simulink model "PneumaticsSystem"  (R2019b)
settings: configuration reference "ConfigSet_PneumaticsSystem_Reference" (kept outside this file)
PostLoadFcn:
  | set_up_test_model()
model workspace (MAT data in the model file):
  PAtm = 101300
  Prm_PneumaticsSystem = Simulink.Parameter
  Prm_PneumaticsSystem.Value.BrakeControl.LoadCompensationGains = [0.66 1]
  Prm_PneumaticsSystem.Value.BrakeControl.MaxPressure = 443000
  Prm_PneumaticsSystem.Value.MainReservoir.ResetPressure = 1000000
  Prm_PneumaticsSystem.Value.MainReservoir.MaxPressure = 1200000
  Prm_PneumaticsSystem.Value.MainReservoir.Volume = 0.2
  Prm_PneumaticsSystem.Value.MainReservoir.SwitchONPressure = 1000000
  Prm_PneumaticsSystem.Value.MainReservoir.SwitchOFFPressure = 750000
  Prm_PneumaticsSystem.Value.MainReservoir.CompressorMassFlowRate = 0.022
  Prm_PneumaticsSystem.Value.MainReservoir.BlowOffONPressure = 1050000
  Prm_PneumaticsSystem.Value.MainReservoir.BlowOffOFFPressure = 1000000
  Prm_PneumaticsSystem.Value.MainReservoirPipe.ResetPressure = 1000000
  Prm_PneumaticsSystem.Value.MainReservoirPipe.SwitchONPressure = 1000000
  Prm_PneumaticsSystem.Value.MainReservoirPipe.SwitchOFFPressure = 750000
  Prm_PneumaticsSystem.Value.Sanding.SwitchONPressure = 380000
  Prm_PneumaticsSystem.Value.Sanding.SwitchOFFPressure = 360000
  Prm_PneumaticsSystem.Value.AirSuspension.LoadCompensationMasses = [21000 33350]
  Prm_PneumaticsSystem.Value.AirSuspension.LoadCompensationPressures = [165000 440000]
  Prm_PneumaticsSystem.Value.AirSuspension.MaxPressure = 510000
  Prm_PneumaticsSystem.Value.AirSuspension.Volume = 0.07
  Prm_PneumaticsSystem.Value.AirSuspension.SwitchONPressure = 220000
  Prm_PneumaticsSystem.Value.AirSuspension.SwitchOFFPressure = 180000
  Prm_PneumaticsSystem.Value.Horn.SwitchONPressure = 140000
  Prm_PneumaticsSystem.Value.AuxiliaryReservoir.ResetPressure = 1000000
  Prm_PneumaticsSystem.Value.AuxiliaryReservoir.MaxPressure = 1000000
  Prm_PneumaticsSystem.Value.AuxiliaryReservoir.Volume = 0.025
  Prm_PneumaticsSystem.Value.AuxiliaryReservoir.SwitchONPressure = 700000
  Prm_PneumaticsSystem.Value.AuxiliaryReservoir.SwitchOFFPressure = 600000
  Prm_PneumaticsSystem.Value.AuxiliaryReservoir.CompressorMassFlowRate = 0.0014
  Prm_PneumaticsSystem.Value.AuxiliaryReservoir.BlowOffONPressure = 1020000
  Prm_PneumaticsSystem.Value.AuxiliaryReservoir.BlowOffOFFPressure = 1000000
  Prm_PneumaticsSystem.Value.Pantograph.ResetPressure = 0
  Prm_PneumaticsSystem.Value.Pantograph.MaxPressure = 1000000
  Prm_PneumaticsSystem.Value.Pantograph.Volume = 0.003
  Prm_PneumaticsSystem.Value.Pantograph.SwitchONPressure = 380000
  Prm_PneumaticsSystem.Value.Pantograph.SwitchOFFPressure = 280000
  Prm_PneumaticsSystem.Value.Pantograph.ORDSwitchONPressure = 300000
  Prm_PneumaticsSystem.Value.Pantograph.ORDSwitchOFFPressure = 240000
  Prm_PneumaticsSystem.Value.BrakeReservoir.ResetPressure = 1000000
  Prm_PneumaticsSystem.Value.BrakeReservoir.MaxPressure = 1200000
  Prm_PneumaticsSystem.Value.BrakeReservoir.Volume = 0.1
  Prm_PneumaticsSystem.Value.BrakeReservoir.SwitchONPressure = 650000
  Prm_PneumaticsSystem.Value.BrakeReservoir.SwitchOFFPressure = 550000
  Prm_PneumaticsSystem.Value.BrakeCylinder.BrakeCylindersPerBogieAxle = [2 2]
  Prm_PneumaticsSystem.Value.BrakeCylinder.ResetPressure = 0
  Prm_PneumaticsSystem.Value.BrakeCylinder.MaxPressure = 600000
  Prm_PneumaticsSystem.Value.BrakeCylinder.Volume = 0.0125
  Prm_PneumaticsSystem.Value.BrakeCylinder.SwitchONPressure = 60000
  Prm_PneumaticsSystem.Value.BrakeCylinder.SwitchOFFPressure = 30000
  Prm_PneumaticsSystem.Value.ParkBrakes.ParkBrakesPerBogieAxle = [1 1]
  Prm_PneumaticsSystem.Value.ParkBrakes.ParkBrakePressures = [300000 480000]
  Prm_PneumaticsSystem.Value.ParkBrakes.ParkBrakeForces = [31500 0]
  Prm_PneumaticsSystem.Value.ParkBrakes.SwitchONPressure = 480000
  Prm_PneumaticsSystem.Value.ParkBrakes.SwitchOFFPressure = 380000
  Prm_PneumaticsSystem.Value.VCB.ResetPressure = 0
  Prm_PneumaticsSystem.Value.VCB.MaxPressure = 1000000
  Prm_PneumaticsSystem.Value.VCB.Volume = 0.0005
  Prm_PneumaticsSystem.Value.VCB.SwitchONPressure = 435000
  Prm_PneumaticsSystem.Value.VCB.SwitchOFFPressure = 385000
  Prm_PneumaticsSystem.DataType = 'Bus: BD_PneumaticsSystem_Prm'
  Prm_PneumaticsSystem.Dimensions = [1 1]
  SampleTime = 0.01
undefined symbols (not defined in the file): AirSuspensionBogie1Deflated, AirSuspensionPressure, AirSuspensionPressureSwitch, AirSuspPressureDiff, AuxiliaryReservoirPressure, AuxiliaryReservoirPressureSwitch, BECU1BrakeNotApplied, BECU1BrakeNotReleased, BECU1CarLoadPressureLow, BECU1EmergencyBrakeFailure, BECU1LoadPressureLow, BECU1ServiceBrakeFailure, BECU2CarLoadPressureLow, BECU2EmergencyBrakeFailure, BECULowRPressure, Bogie, BrakeCylinderControlPressure, BrakeCylinderPressure, BrakeCylinderPressureGauge, BrakeCylinderPressureSwitch, BrakeReservoirPressure, BrakeReservoirPressureSwitch, HornHighPressureSwitch, HornLowPressureSwitch, MainReservoirPipePressure, MainReservoirPipePressureSwitch, MainReservoirPressure, MainReservoirPressureGauge, MainReservoirPressureSwitch, MaxAxles, MRPS_TractionCutout, ORDPressureSwitch, PantographCylinderPressure, ParkBrakePressure, ParkBrakePressureGauge, ParkBrakePressureSwitch, PS2, PS3, SandingSystemPressure, SandingSystemPressureSwitch, SRPressureGauge, VCBCylinderPressure, VCBPressureSwitch
libraries: PneumaticLib x56, simulink x50, LatchesLib x7, FiltersLib x4, TimersLib x3, MathOperationsLib x3, VectorOperationsLib x1, simulink_extras x1
(part 1 of 3)
settings Model: PauseTimes=3  ParameterArgumentNames=Prm_PneumaticsSystem  Creator=cdyer  LastModifiedBy=hinganes
settings ConfigSetRef: SourceName=ConfigSet_PneumaticsSystem_Reference  SourceLocation=Base Workspace

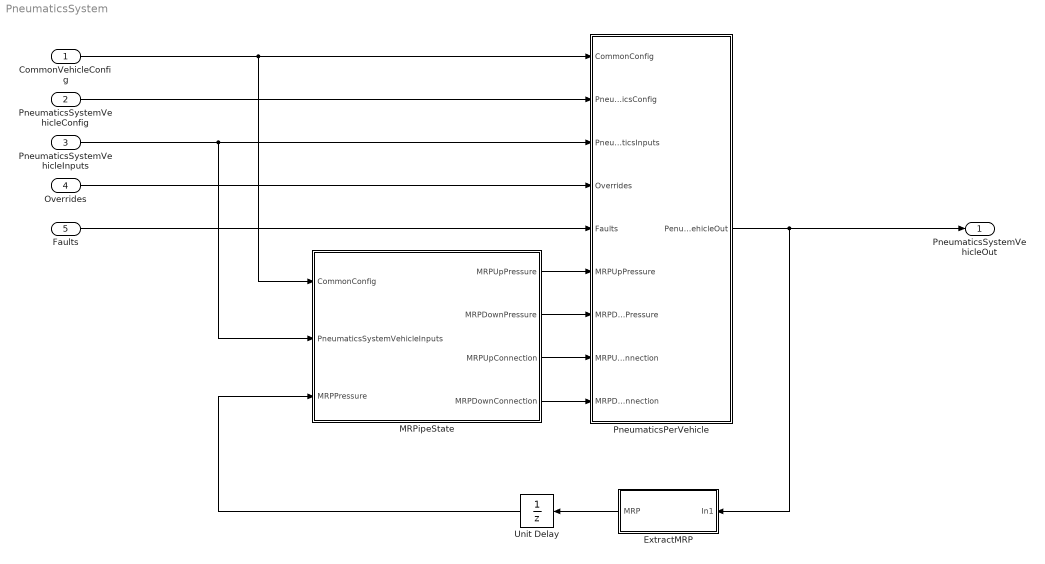
== system PneumaticsSystem ==
  CommonVehicleConfig : Inport  OutDataTypeStr=Bus: BD_CommonTrain_Cfg_Vehicle  PortDimensions=MaxVehicles  BusOutputAsStruct=on
  PneumaticsSystemVehicleConfig : Inport  Port=2  OutDataTypeStr=Bus: BD_PneumaticsSystem_Cfg_Vehicle  PortDimensions=MaxVehicles  BusOutputAsStruct=on
  PneumaticsSystemVehicleInputs : Inport  Port=3  OutDataTypeStr=Bus: BD_PneumaticsSystem_In_Vehicle  PortDimensions=MaxVehicles  BusOutputAsStruct=on
  Overrides : Inport  Port=4  OutDataTypeStr=Bus: BD_PneumaticsSystem_In_Overrides  BusOutputAsStruct=on
  Faults : Inport  Port=5  OutDataTypeStr=Bus: BD_PneumaticsSystem_In_Vehicle_Faults  BusOutputAsStruct=on
  ExtractMRP : Subsystem  TreatAsAtomicUnit=on
  MRPipeState : Subsystem
  PneumaticsPerVehicle : Subsystem
  Unit Delay : UnitDelay  SampleTime=-1  HasFrameUpgradeWarning=on
  PneumaticsSystemVehicleOut : Outport  OutDataTypeStr=Bus: BD_PneumaticsSystem_Out_Vehicle  BusOutputAsStruct=on
  wires:
  Faults/1 -> PneumaticsPerVehicle/5(Faults)
  PneumaticsSystemVehicleInputs/1 -> PneumaticsPerVehicle/3(PneumaticsInputs), MRPipeState/2(PneumaticsSystemVehicleInputs)
  Overrides/1 -> PneumaticsPerVehicle/4(Overrides)
  PneumaticsPerVehicle/1(PenumaticsVehicleOut) -> PneumaticsSystemVehicleOut/1, ExtractMRP/1(In1)
  ExtractMRP/1(MRP) -> Unit Delay/1
  Unit Delay/1 -> MRPipeState/3(MRPPressure)
  MRPipeState/1(MRPUpPressure) -> PneumaticsPerVehicle/6(MRPUpPressure)
  MRPipeState/2(MRPDownPressure) -> PneumaticsPerVehicle/7(MRPDownPressure)
  MRPipeState/3(MRPUpConnection) -> PneumaticsPerVehicle/8(MRPUpConnection)
  CommonVehicleConfig/1 -> MRPipeState/1(CommonConfig), PneumaticsPerVehicle/1(CommonConfig)
  PneumaticsSystemVehicleConfig/1 -> PneumaticsPerVehicle/2(PneumaticsConfig)
  MRPipeState/4(MRPDownConnection) -> PneumaticsPerVehicle/9(MRPDownConnection)

== system PneumaticsSystem/ExtractMRP ==
  In1 : Inport  Partition=on  PartitionDimension=1  PartitionWidth=1  PartitionOffset=0
  Bus Selector1 : BusSelector  OutputSignals=Debug.MainReservoirPipePressure
  For Each : ForEach  DisableCoverage=on
  MRP : Outport  ConcatenationDimension=1
  wires:
  In1/1 -> Bus Selector1/1
  Bus Selector1/1 -> MRP/1  "<MainReservoirPipePressure>"

== system PneumaticsSystem/MRPipeState ==
  CommonConfig : Inport
  PneumaticsSystemVehicleInputs : Inport  Port=2
  MRPPressure : Inport  Port=3
  Extract : Subsystem  TreatAsAtomicUnit=on
  Head : Selector  NumberOfDimensions=2  InputPortWidth=3  IndexOptions=Select all,Index vector (dialog)  Indices=[1],[1]  OutputSizes=1,1
  Orientation Swap : VectorOperationsLib/Orientation Swap
      settings: SourceProductName=Sydac Utilities
  PipeConnections : MATLAB Function  TreatAsAtomicUnit=on
  Product : Product
  Product1 : Product
  Tail : Selector  NumberOfDimensions=2  InputPortWidth=3  IndexOptions=Select all,Index vector (dialog)  Indices=[1],[2]  OutputSizes=1,1
  UpDnSel : MATLAB Function  TreatAsAtomicUnit=on
  MRPUpPressure : Outport
  MRPDownPressure : Outport  Port=2
  MRPUpConnection : Outport  Port=3
  MRPDownConnection : Outport  Port=4
  wires:
  UpDnSel/2(yDn) -> MRPDownPressure/1
  MRPPressure/1 -> UpDnSel/1(u)
  UpDnSel/1(yUp) -> MRPUpPressure/1
  PipeConnections/2(rearState) -> MRPDownConnection/1
  PipeConnections/1(frontState) -> MRPUpConnection/1
  PneumaticsSystemVehicleInputs/1 -> Extract/2(PneumaticsSystemVehicleInputs)
  CommonConfig/1 -> Extract/1(CommonConfig)
  Extract/4(Orientation) -> Orientation Swap/3
  Orientation Swap/1 -> PipeConnections/1(frontCock)  "Front"
  Orientation Swap/2 -> PipeConnections/2(rearCock)  "Rear"
  Product/1 -> Orientation Swap/1
  Product1/1 -> Orientation Swap/2
  Extract/1(Enabled) -> Product1/1, Product/1
  Extract/2(End1Cock) -> Product/2
  Extract/3(End2Cock) -> Product1/2
  Head/1 -> PipeConnections/3(frontCoupled)  "Front"
  Tail/1 -> PipeConnections/4(rearCoupled)  "Rear"
  Extract/5(PneumaticCouplingState) -> Tail/1, Head/1

== system PneumaticsSystem/PneumaticsPerVehicle ==
  CommonConfig : Inport  Partition=on  PartitionDimension=1  PartitionWidth=1  PartitionOffset=0
  PneumaticsConfig : Inport  Port=2  Partition=on  PartitionDimension=1  PartitionWidth=1  PartitionOffset=0
  PneumaticsInputs : Inport  Port=3  Partition=on  PartitionDimension=1  PartitionWidth=1  PartitionOffset=0
  Overrides : Inport  Port=4  Partition=on  PartitionDimension=1  PartitionWidth=1  PartitionOffset=0
  Faults : Inport  Port=5  Partition=on  PartitionDimension=1  PartitionWidth=1  PartitionOffset=0
  MRPUpPressure : Inport  Port=6  Partition=on  PartitionDimension=1  PartitionWidth=1  PartitionOffset=0
  MRPDownPressure : Inport  Port=7  Partition=on  PartitionDimension=1  PartitionWidth=1  PartitionOffset=0
  MRPUpConnection : Inport  Port=8  Partition=on  PartitionDimension=1  PartitionWidth=1  PartitionOffset=0
  MRPDownConnection : Inport  Port=9  Partition=on  PartitionDimension=1  PartitionWidth=1  PartitionOffset=0
  Bus Selector : BusSelector  OutputSignals=Enabled
  For Each : ForEach  DisableCoverage=on
  PneumaticsSystem : Subsystem
  PenumaticsVehicleOut : Outport  ConcatenationDimension=1
  wires:
  CommonConfig/1 -> PneumaticsSystem/1(CommonConfig), Bus Selector/1
  PneumaticsInputs/1 -> PneumaticsSystem/3(PneumaticsInputs)
  Overrides/1 -> PneumaticsSystem/4(Overrides)
  Faults/1 -> PneumaticsSystem/5(Faults)
  MRPUpPressure/1 -> PneumaticsSystem/6(MRPUpPressure)
  MRPDownPressure/1 -> PneumaticsSystem/7(MRPDownPressure)
  MRPUpConnection/1 -> PneumaticsSystem/8(MRPUpConnection)
  MRPDownConnection/1 -> PneumaticsSystem/9(MRPDownConnection)
  PneumaticsSystem/1(PenumaticsVehicleOut) -> PenumaticsVehicleOut/1
  PneumaticsConfig/1 -> PneumaticsSystem/2(PneumaticsConfig)  "Pneumatics"
  Bus Selector/1 -> PneumaticsSystem/Enable  "<Enabled>"

== system PneumaticsSystem/MRPipeState/Extract ==
  CommonConfig : Inport  Partition=on  PartitionDimension=1  PartitionWidth=1  PartitionOffset=0
  PneumaticsSystemVehicleInputs : Inport  Port=2  Partition=on  PartitionDimension=1  PartitionWidth=1  PartitionOffset=0
  Bus Selector : BusSelector  OutputSignals=InputControlStates.InterCarIsolationCockEnd1,InputControlStates.InterCarIsolationCockEnd2,PhysicalSignals.PneumaticallyCoupled,InputControlStates.UncouplingIsolationCock
  Bus Selector2 : BusSelector  OutputSignals=Orientation,Enabled
  For Each : ForEach  DisableCoverage=on
  Logical Operator : Logic  AllPortsSameDT=off  OutDataTypeStr=boolean
  Reshape : Reshape  OutputDimensionality=Row vector (2-D)
  Enabled : Outport  ConcatenationDimension=1
  End1Cock : Outport  Port=2  ConcatenationDimension=1
  End2Cock : Outport  Port=3  ConcatenationDimension=1
  Orientation : Outport  Port=4  ConcatenationDimension=1
  PneumaticCouplingState : Outport  Port=5  ConcatenationDimension=1
  wires:
  CommonConfig/1 -> Bus Selector2/1
  Bus Selector2/1 -> Orientation/1  "<Orientation>"
  Bus Selector2/2 -> Enabled/1  "<Enabled>"
  PneumaticsSystemVehicleInputs/1 -> Bus Selector/1
  Bus Selector/1 -> End1Cock/1  "<InterCarIsolationCockEnd1>"
  Bus Selector/2 -> End2Cock/1  "<InterCarIsolationCockEnd2>"
  Bus Selector/3 -> Logical Operator/1  "<PneumaticallyCoupled>"
  Reshape/1 -> PneumaticCouplingState/1
  Bus Selector/4 -> Logical Operator/2  "<UncouplingIsolationCock>"
  Logical Operator/1 -> Reshape/1

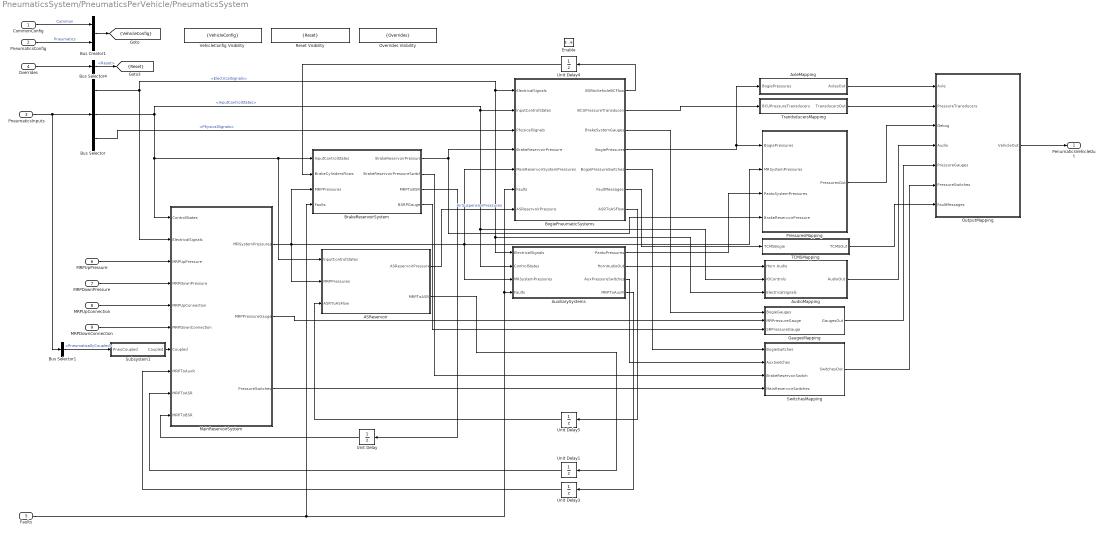
== system PneumaticsSystem/PneumaticsPerVehicle/PneumaticsSystem ==
  CommonConfig : Inport
  PneumaticsConfig : Inport  Port=2
  PneumaticsInputs : Inport  Port=3
  Overrides : Inport  Port=4
  Faults : Inport  Port=5
  MRPUpPressure : Inport  Port=6
  MRPDownPressure : Inport  Port=7
  MRPUpConnection : Inport  Port=8
  MRPDownConnection : Inport  Port=9
  Enable : EnablePort
  ASReservoir : Subsystem
  AudioMapping : Subsystem
  AuxiliarySystems : Subsystem
  AxleMapping : Subsystem
  BogiePneumaticSystems : Subsystem
  BrakeReservoirSystem : Subsystem
  Bus Creator1 : BusCreator  Inputs=2
  Bus Selector : BusSelector  OutputSignals=ElectricalSignals,InputControlStates,PhysicalSignals
  Bus Selector1 : BusSelector  OutputSignals=PhysicalSignals.PneumaticallyCoupled
  Bus Selector4 : BusSelector  OutputSignals=Reset
  GaugesMapping : Subsystem
  MainReservoirSystem : Subsystem
  OutputMapping : Subsystem
  Overrides Visibility : GotoTagVisibility  GotoTag=Overrides
  PressuresMapping : Subsystem
  Reset Visibility : GotoTagVisibility  GotoTag=Reset
  Subsystem1 : Subsystem
  SwitchesMapping : Subsystem
  TCMSMapping : Subsystem
  TrandsducersMapping : Subsystem
  Unit Delay{,1,3..5} (5 alike) : UnitDelay  SampleTime=-1  HasFrameUpgradeWarning=on
  VehicleConfig Visibility : GotoTagVisibility  GotoTag=VehicleConfig
  PenumaticsVehicleOut : Outport
  tag scope: Reset=scoped, VehicleConfig=scoped
  wires:
  Overrides/1 -> Bus Selector4/1
  OutputMapping/1(VehicleOut) -> PenumaticsVehicleOut/1
  AuxiliarySystems/1(PantoPressures) -> PressuresMapping/3(PantoSystemPressures)
  PneumaticsInputs/1 -> Bus Selector1/1, Bus Selector/1
  Bus Selector/1 -> AudioMapping/3(ElectricalSignals), AuxiliarySystems/1(ElectricalSignals), BogiePneumaticSystems/1(ElectricalSignals), MainReservoirSystem/2(ElectricalSignals)  "<ElectricalSignals>"
  Bus Selector/2 -> AudioMapping/2(IOControls), AuxiliarySystems/2(ControlStates), BogiePneumaticSystems/2(InputControlStates), MainReservoirSystem/1(ControlStates), ASReservoir/1(InputControlStates), BrakeReservoirSystem/1(InputControlStates)  "<InputControlStates>"
  Unit Delay/1 -> MainReservoirSystem/10(MRPToBSR)
  MRPUpPressure/1 -> MainReservoirSystem/3(MRPUpPressure)
  MRPDownPressure/1 -> MainReservoirSystem/4(MRPDownPressure)
  MRPUpConnection/1 -> MainReservoirSystem/5(MRPUpConnection)
  MRPDownConnection/1 -> MainReservoirSystem/6(MRPDownConnection)
  MainReservoirSystem/2(MRPPressureGauge) -> GaugesMapping/2(MRPressureGauge)
  PressuresMapping/1(PressuresOut) -> OutputMapping/3(Debug)
  GaugesMapping/1(GaugesOut) -> OutputMapping/5(PressureGauges)
  SwitchesMapping/1(SwitchesOut) -> OutputMapping/6(PressureSwitches)
  AudioMapping/1(AudioOut) -> OutputMapping/4(Audio)
  TrandsducersMapping/1(TransducersOut) -> OutputMapping/2(PressureTransducers)
  BrakeReservoirSystem/1(BrakeReservoirPressure) -> BogiePneumaticSystems/4(BrakeReservoirPressure), PressuresMapping/4(BrakeReservoirPressure)
  MainReservoirSystem/3(PressureSwitches) -> SwitchesMapping/4(MainReservoirSwitches)
  PneumaticsConfig/1 -> Bus Creator1/2  "Pneumatics"
  Bus Creator1/1 -> [VehicleConfig]
  Bus Selector4/1 -> [Reset]  "<Reset>"
  Bus Selector/3 -> BogiePneumaticSystems/3(PhysicalSignals)  "<PhysicalSignals>"
  AuxiliarySystems/2(HornAudioOut) -> AudioMapping/1(Horn Audio)
  AuxiliarySystems/3(AuxPressureSwitches) -> SwitchesMapping/2(AuxSwitches)
  Unit Delay3/1 -> MainReservoirSystem/8(MRPToAuxR)
  BogiePneumaticSystems/2(BCUPressureTransducers) -> TrandsducersMapping/1(BCUPressureTransducers)
  BogiePneumaticSystems/3(BrakeSystemGauges) -> GaugesMapping/1(BogieGauges)
  BogiePneumaticSystems/4(BogiePressures) -> AxleMapping/1(BogiePressures), PressuresMapping/1(BogiePressures)
  BogiePneumaticSystems/5(BogiePressureSwitches) -> SwitchesMapping/1(BogieSwitches)
  MainReservoirSystem/1(MRSystemPressures) -> BrakeReservoirSystem/3(MRPPressures), ASReservoir/2(MRPPressures), BogiePneumaticSystems/5(MainReservoirSystemPressures), PressuresMapping/2(MRSystemPressures), AuxiliarySystems/3(MRSystemPressures)
  BogiePneumaticSystems/1(BSRtoVehicleBCFlow) -> Unit Delay4/1
  Unit Delay4/1 -> BrakeReservoirSystem/2(BrakeCylindersFlows)
  ASReservoir/1(ASReservoirPressure) -> BogiePneumaticSystems/7(ASReservoirPressure)  "AirSuspensionPressures"
  BrakeReservoirSystem/2(BrakeReservoirPressureSwitch) -> SwitchesMapping/3(BrakeReservoirSwitch)
  CommonConfig/1 -> Bus Creator1/1  "Common"
  AxleMapping/1(AxlesOut) -> OutputMapping/1(Axle)
  Faults/1 -> BrakeReservoirSystem/4(Faults), BogiePneumaticSystems/6(Faults), AuxiliarySystems/4(Faults)
  BogiePneumaticSystems/6(FaultMessages) -> TCMSMapping/1(TCMSBogie)
  TCMSMapping/1(TCMSOut) -> OutputMapping/7(FaultMessages)
  Unit Delay1/1 -> MainReservoirSystem/9(MRPToASR)
  BogiePneumaticSystems/7(ASRToASFlow) -> Unit Delay5/1
  Unit Delay5/1 -> ASReservoir/3(ASRToASFlow)
  ASReservoir/2(MRPToASR) -> Unit Delay1/1
  BrakeReservoirSystem/3(MRPToBSR) -> Unit Delay/1
  BrakeReservoirSystem/4(BSRPGauge) -> GaugesMapping/3(SRPressureGauge)
  AuxiliarySystems/4(MRPToAuxR) -> Unit Delay3/1
  Bus Selector1/1 -> Subsystem1/1(PneuCoupled)  "<PneumaticallyCoupled>"
  Subsystem1/1(Coupled) -> MainReservoirSystem/7(Coupled)

== system PneumaticsSystem/PneumaticsPerVehicle/PneumaticsSystem/ASReservoir ==
  InputControlStates : Inport
  MRPPressures : Inport  Port=2
  ASRToASFlow : Inport  Port=3
  Air SuspensionReservoir : Subsystem  mask{ResetPressure=9e5, MaxPressure=10e5, Volume=0.05}
      mask prompts: ResetPressure "Reset Pressure [Pa]"; MaxPressure "Max Pressure [Pa]"; Volume "Reservoir Volume [m^3]"
  Bus Selector1 : BusSelector  OutputSignals=MainReservoirPipePressure
  Bus Selector3 : BusSelector  OutputSignals=AirSuspensionReservoirIsolationCock
  Constant : Constant  Value=0
  Ground : Ground
  ASReservoirPressure : Outport
  MRPToASR : Outport  Port=2
  wires:
  Bus Selector1/1 -> Air SuspensionReservoir/1(MRPPressure)  "<MainReservoirPipePressure>"
  Ground/1 -> Air SuspensionReservoir/7(PresetVal), Air SuspensionReservoir/6(Preset)
  InputControlStates/1 -> Bus Selector3/1
  [Reset] -> Air SuspensionReservoir/5(Reset)
  Bus Selector3/1 -> Air SuspensionReservoir/2(ASRIsolCock)  "<AirSuspensionReservoirIsolationCock>"
  Air SuspensionReservoir/1(ASPressure) -> ASReservoirPressure/1  "ASReservoirPressure"
  MRPPressures/1 -> Bus Selector1/1
  Constant/1 -> Air SuspensionReservoir/3(ASRDrainCock)
  ASRToASFlow/1 -> Air SuspensionReservoir/4(ASFlow)
  Air SuspensionReservoir/2(MRPToASR) -> MRPToASR/1

== system PneumaticsSystem/PneumaticsPerVehicle/PneumaticsSystem/AudioMapping ==
  Horn Audio : Inport
  IOControls : Inport  Port=2
  ElectricalSignals : Inport  Port=3
  Brake Supply Reservoir Pressure available : Constant
  Bus Creator : BusCreator  Inputs=4
  Bus Selector : BusSelector  OutputSignals=NoEmergencyBrakeValve
  Bus Selector2 : BusSelector  OutputSignals=HornLow,HornHigh
  Data Type Conversion : DataTypeConversion
  Data Type Conversion1 : DataTypeConversion
  Detect Decrease : simulink/Logic and Bit Operations/Detect Decrease  vinit=0.0  OutDataTypeStr=boolean
  Logical Operator1 : Logic  AllPortsSameDT=off  OutDataTypeStr=boolean
  Subsystem : Subsystem
  TimerOffDelay NoInit : TimersLib/TimerOffDelay NoInit  UpperSaturationLimit=1  SampleTime=-1
      settings: SourceProductName=Sydac Utilities
  TimerOffDelay NoInit1 : TimersLib/TimerOffDelay NoInit  UpperSaturationLimit=1  SampleTime=-1
      settings: SourceProductName=Sydac Utilities
  AudioOut : Outport
  wires:
  Bus Selector2/2 -> Bus Creator/2  "<HornHigh>"
  Bus Creator/1 -> AudioOut/1  "Audio"
  Bus Selector2/1 -> Bus Creator/1  "<HornLow>"
  Horn Audio/1 -> Bus Selector2/1
  Subsystem/1(ReleaseAudio) -> TimerOffDelay NoInit1/1
  Logical Operator1/1 -> TimerOffDelay NoInit/1
  Data Type Conversion/1 -> Bus Creator/3  "PneumaticPressureRelease"
  Data Type Conversion1/1 -> Bus Creator/4  "EmergencyBrakeActive"
  IOControls/1 -> Subsystem/1(IsolationCocks)
  Brake Supply Reservoir Pressure available/1 -> Logical Operator1/1
  ElectricalSignals/1 -> Bus Selector/1
  Bus Selector/1 -> Detect Decrease/1  "<NoEmergencyBrakeValve>"
  Detect Decrease/1 -> Logical Operator1/2
  TimerOffDelay NoInit/1 -> Data Type Conversion1/1
  TimerOffDelay NoInit1/1 -> Data Type Conversion/1

== system PneumaticsSystem/PneumaticsPerVehicle/PneumaticsSystem/AuxiliarySystems ==
  ElectricalSignals : Inport
  ControlStates : Inport  Port=2
  MRSystemPressures : Inport  Port=3
  Faults : Inport  Port=4
  AuxSystem : Subsystem
  Bus Creator : BusCreator  Inputs=2
  Bus Selector : BusSelector  OutputSignals=Pneumatics.Equipment.HasPantograph
  Bus Selector1 : BusSelector  OutputSignals=Pneumatics.Equipment.HasDriverCab
  Bus Selector2 : BusSelector  OutputSignals=MainReservoirPipePressure
  Horn : Subsystem  mask{PressureSwitchON=Prm_PneumaticsSystem.Horn.SwitchONPressure}
      mask prompts: PressureSwitchON "Air Supply Pressure Switch ON Point [Pa]"
  PantoPressures : Outport
  HornAudioOut : Outport  Port=2
  AuxPressureSwitches : Outport  Port=3
  MRPToAuxR : Outport  Port=4
  wires:
  Horn/1(PressureSwitches) -> Bus Creator/2
  Horn/2(AudioOut) -> HornAudioOut/1
  AuxSystem/2(PressureSwitches) -> Bus Creator/1
  ElectricalSignals/1 -> Horn/3(ElectricalSignals), AuxSystem/2(ElectricalSignals)
  AuxSystem/1(PantoSystemPressures) -> PantoPressures/1
  MRSystemPressures/1 -> Bus Selector2/1, AuxSystem/3(MRSystemPressures)
  ControlStates/1 -> Horn/1(ControlStates), AuxSystem/1(ControlStates)
  Bus Creator/1 -> AuxPressureSwitches/1
  [VehicleConfig] -> Bus Selector/1
  Bus Selector/1 -> AuxSystem/Enable  "<HasPantograph>"
  Bus Selector1/1 -> Horn/Enable  "<HasDriverCab>"
  [Reset] -> AuxSystem/5(Reset)
  [VehicleConfig] -> Bus Selector1/1
  Bus Selector2/1 -> Horn/2(HornSupplyPressure)  "<MainReservoirPipePressure>"
  Faults/1 -> AuxSystem/4(Faults)
  AuxSystem/3(MRPToAuxR) -> MRPToAuxR/1

== system PneumaticsSystem/PneumaticsPerVehicle/PneumaticsSystem/AxleMapping ==
  BogiePressures : Inport
  Assignment : Assignment  DiagnosticForDimensions=Warning  IndexOptions=Starting index (dialog)  Indices=1  OutputSizes=1
  Assignment1 : Assignment  DiagnosticForDimensions=Warning  IndexOptions=Starting index (dialog)  Indices=3  OutputSizes=1
  Assignment2 : Assignment  DiagnosticForDimensions=Warning  IndexOptions=Index vector (dialog)  Indices=[1 2]  OutputSizes=1
  Assignment3 : Assignment  DiagnosticForDimensions=Warning  IndexOptions=Index vector (dialog)  Indices=[3 4]  OutputSizes=1
  Bogie1 : Selector  InputPortWidth=2  IndexOptions=Index vector (dialog)  Indices=1  OutputSizes=1
  Bogie2 : Selector  InputPortWidth=2  IndexOptions=Index vector (dialog)  Indices=2  OutputSizes=1
  Bus Creator : BusCreator  Inputs=2  OutDataTypeStr=Bus: BD_PneumaticsSystem_Out_Vehicle_AxleBrakes  NonVirtualBus=on
  Bus Selector : BusSelector  OutputSignals=BrakeCylinderPressure,ParkBrakePressure
  Bus Selector1 : BusSelector  OutputSignals=BrakeCylinderPressure,ParkBrakePressure
  Constant : Constant  Value=zeros(1,MaxAxles)
  AxlesOut : Outport
  wires:
  BogiePressures/1 -> Bogie1/1, Bogie2/1  "Bogie"
  Bogie1/1 -> Bus Selector/1
  Bogie2/1 -> Bus Selector1/1
  Bus Selector/1 -> Assignment/2  "<BrakeCylinderPressure>"
  Bus Selector1/1 -> Assignment1/2  "<BrakeCylinderPressure>"
  Constant/1 -> Assignment2/1, Assignment/1
  Assignment/1 -> Assignment1/1
  Bus Selector/2 -> Assignment2/2  "<ParkBrakePressure>"
  Assignment2/1 -> Assignment3/1
  Bus Selector1/2 -> Assignment3/2  "<ParkBrakePressure>"
  Assignment1/1 -> Bus Creator/1  "BrakeCylinderPressures"
  Assignment3/1 -> Bus Creator/2  "ParkBrakePressures"
  Bus Creator/1 -> AxlesOut/1  "AxleBrakes"

== system PneumaticsSystem/PneumaticsPerVehicle/PneumaticsSystem/BogiePneumaticSystems ==
  ElectricalSignals : Inport
  InputControlStates : Inport  Port=2
  PhysicalSignals : Inport  Port=3
  BrakeReservoirPressure : Inport  Port=4
  MainReservoirSystemPressures : Inport  Port=5
  Faults : Inport  Port=6
  ASReservoirPressure : Inport  Port=7
  AirSuspensionSystem : Subsystem  mask{LoadCompensationMasses=Prm_PneumaticsSystem.AirSuspension.LoadCompensationMasses, LoadCompensationPressures=Prm_PneumaticsSystem.AirSuspension.LoadCompensationPressures, MaxPressure=Prm_PneumaticsSystem.AirSuspension.MaxPressure, Volume=Prm_PneumaticsSystem.AirSuspension.Volume, PressureSwitchON=Prm_PneumaticsSystem.AirSuspension.SwitchONPressure, PressureSwitchOFF=Prm_PneumaticsSystem.AirSuspension.SwitchOFFPressure}
      mask prompts: LoadCompensationMasses "Load Compensation Masses [kg]"; LoadCompensationPressures "Load Compensation Pressures [Pa]"; MaxPressure "Max Pressure [Pa]"; Volume "Reservoir Volume [m^3]"; PressureSwitchON "Pressure Switch ON Point [Pa]"; PressureSwitchOFF "Pressure Switch OFF Point [Pa]"
  BogiePressureMapping : Subsystem  TreatAsAtomicUnit=on
  BogiePressureSwitchesMapping : Subsystem  TreatAsAtomicUnit=on
  BrakingSystem : Subsystem
  Bus Selector1 : BusSelector  OutputSignals=MainReservoirPipePressure
  Bus Selector3 : BusSelector  OutputSignals=Pneumatics.Equipment.HasBogie
  SandingSystem : Subsystem  mask{PressureSwitchON=Prm_PneumaticsSystem.Sanding.SwitchONPressure, PressureSwitchOFF=Prm_PneumaticsSystem.Sanding.SwitchOFFPressure}
      mask prompts: PressureSwitchON "Pressure Switch ON Point [Pa]"; PressureSwitchOFF "Pressure Switch OFF Point [Pa]"
  BSRtoVehicleBCFlow : Outport
  BCUPressureTransducers : Outport  Port=2
  BrakeSystemGauges : Outport  Port=3
  BogiePressures : Outport  Port=4
  BogiePressureSwitches : Outport  Port=5
  FaultMessages : Outport  Port=6
  ASRToASFlow : Outport  Port=7
  wires:
  BrakingSystem/3(BrakeSystemGauges) -> BrakeSystemGauges/1  "BrakeSystemGauges"
  BrakingSystem/5(BrakeCylinderPressures) -> BogiePressureMapping/2(BrakeCylinderPressures)  "BrakeCylinderPressures"
  SandingSystem/2(SandingPressureSwitches) -> BogiePressureSwitchesMapping/4(SandingPressureSwitches)  "SandingPressureSwitches"
  AirSuspensionSystem/1(AirSuspensionPressure) -> BogiePressureMapping/4(AirSuspensionPressures), BrakingSystem/5(AirSuspensionPresures)  "AirSuspensionPressures"
  BrakingSystem/2(BCUPressureTransducers) -> BCUPressureTransducers/1  "BCUPressureTransducers"
  BrakingSystem/7(BrakeCylinderPressureSwitches) -> BogiePressureSwitchesMapping/1(BrakeCylinderPressureSwitches)  "BrakeSystemPressureSwitches"
  AirSuspensionSystem/2(ASPressureSwitches) -> BogiePressureSwitchesMapping/3(AirSuspensionPressureSwitches)  "ASPressureSwitches"
  [Reset] -> AirSuspensionSystem/5(Reset)
  Bus Selector3/1 -> SandingSystem/Enable, AirSuspensionSystem/Enable, BrakingSystem/Enable  "<HasBogie>"
  [VehicleConfig] -> Bus Selector3/1
  PhysicalSignals/1 -> AirSuspensionSystem/3(PhysicalSignals)
  Bus Selector1/1 -> SandingSystem/3(SandingSystemSupplyPressure)  "<MainReservoirPipePressure>"
  SandingSystem/1(SandingPressures) -> BogiePressureMapping/5(SandingPressures)  "SandingPressure"
  MainReservoirSystemPressures/1 -> Bus Selector1/1, BrakingSystem/3(MRSystemPressures)
  InputControlStates/1 -> SandingSystem/2(ControlStates), AirSuspensionSystem/2(ControlStates), BrakingSystem/2(ControlStates)
  ElectricalSignals/1 -> SandingSystem/1(ElectricalSignals), BrakingSystem/1(ElectricalSignals)
  [Reset] -> BrakingSystem/6(Reset)
  BrakeReservoirPressure/1 -> BrakingSystem/4(BrakeReservoirPressure)
  BrakingSystem/1(BSRtoVehicleBCFlow) -> BSRtoVehicleBCFlow/1
  BrakingSystem/4(BrakeControlPressures) -> BogiePressureMapping/1(BrakeControlPressures)
  BogiePressureMapping/1(BogiePressures) -> BogiePressures/1
  BrakingSystem/6(ParkBrakePressures) -> BogiePressureMapping/3(ParkBrakePressures)
  BogiePressureSwitchesMapping/1(BogiePressureSwitches) -> BogiePressureSwitches/1
  BrakingSystem/8(ParkBrakePressureSwitches) -> BogiePressureSwitchesMapping/2(ParkBrakePressureSwitches)
  Faults/1 -> AirSuspensionSystem/1(Faults), BrakingSystem/7(PneumaticsFaults)
  BrakingSystem/9(FaultMessages) -> FaultMessages/1
  AirSuspensionSystem/3(AirSuspPressure%Variation) -> BogiePressureMapping/6(AirSuspPressure%Variation), BrakingSystem/8(AirSuspPressureDiff)
  ASReservoirPressure/1 -> AirSuspensionSystem/4(AirSuspensionSupplyPressure)
  AirSuspensionSystem/4(ASRToAS) -> ASRToASFlow/1

== system PneumaticsSystem/PneumaticsPerVehicle/PneumaticsSystem/BrakeReservoirSystem ==
  InputControlStates : Inport
  BrakeCylindersFlows : Inport  Port=2
  MRPPressures : Inport  Port=3
  Faults : Inport  Port=4
  BrakeSupplyReservoir : Subsystem  mask{ResetPressure=Prm_PneumaticsSystem.BrakeReservoir.ResetPressure, MaxPressure=Prm_PneumaticsSystem.BrakeReservoir.MaxPressure, Volume=Prm_PneumaticsSystem.BrakeReservoir.Volume, PressureSwitchON=Prm_PneumaticsSystem.BrakeReservoir.SwitchONPressure, PressureSwitchOFF=Prm_PneumaticsSystem.BrakeReservoir.SwitchOFFPressure}
      mask prompts: ResetPressure "Reset Pressure [Pa]"; MaxPressure "Max Pressure [Pa]"; Volume "Reservoir Volume [m^3]"; PressureSwitchON "Pressure Switch ON Point [Pa]"; PressureSwitchOFF "Pressure Switch OFF Point [Pa]"
  Bus Selector1 : BusSelector  OutputSignals=MainReservoirPipePressure
  Bus Selector2 : BusSelector  OutputSignals=BECULowRPressure
  Bus Selector3 : BusSelector  OutputSignals=BrakeSupplyReservoirIsolationCock,BrakeSupplyReservoirDrainCock
  Bus Selector4 : BusSelector  OutputSignals=Pneumatics.Equipment.HasBrakeSystem
  Ground : Ground
  BrakeReservoirPressure : Outport
  BrakeReservoirPressureSwitch : Outport  Port=2
  MRPToBSR : Outport  Port=3
  BSRPGauge : Outport  Port=4
  wires:
  MRPPressures/1 -> Bus Selector1/1
  BrakeSupplyReservoir/1(BSRPressure) -> BrakeReservoirPressure/1  "BrakeReservoirPressure"
  Bus Selector3/1 -> BrakeSupplyReservoir/2(BSRIsolCock)  "<BrakeSupplyReservoirIsolationCock>"
  BrakeCylindersFlows/1 -> BrakeSupplyReservoir/4(BSRtoBCFlow)
  [Reset] -> BrakeSupplyReservoir/6(Reset)
  InputControlStates/1 -> Bus Selector3/1
  Bus Selector3/2 -> BrakeSupplyReservoir/3(BSRDrainCock)  "<BrakeSupplyReservoirDrainCock>"
  Bus Selector4/1 -> BrakeSupplyReservoir/Enable  "<HasBrakeSystem>"
  [VehicleConfig] -> Bus Selector4/1
  BrakeSupplyReservoir/2(BSRPressureSwitch) -> BrakeReservoirPressureSwitch/1
  Ground/1 -> BrakeSupplyReservoir/7(Preset), BrakeSupplyReservoir/8(PresetVal)
  Bus Selector1/1 -> BrakeSupplyReservoir/1(MRPPressure)  "<MainReservoirPipePressure>"
  Bus Selector2/1 -> BrakeSupplyReservoir/5(LowRPress)  "<BECULowRPressure>"
  Faults/1 -> Bus Selector2/1
  BrakeSupplyReservoir/3(MRPToBSR) -> MRPToBSR/1
  BrakeSupplyReservoir/4(BSRPressureGauge) -> BSRPGauge/1

== system PneumaticsSystem/PneumaticsPerVehicle/PneumaticsSystem/GaugesMapping ==
  BogieGauges : Inport
  MRPressureGauge : Inport  Port=2
  SRPressureGauge : Inport  Port=3
  Bus Assignment : BusAssignment  AssignedSignals=MainReservoirPressureGauge,SRPressureGauge,Bogie
  Constant : Constant  Value=0  OutDataTypeStr=Bus: BD_PneumaticsSystem_Out_Vehicle_Gauges
  Subsystem : Subsystem
  GaugesOut : Outport
  wires:
  Bus Assignment/1 -> GaugesOut/1  "PressureGauges"
  MRPressureGauge/1 -> Bus Assignment/2  "MainReservoirPressureGauge"
  Constant/1 -> Bus Assignment/1
  SRPressureGauge/1 -> Bus Assignment/3  "MainReservoirPressureGauge"
  Subsystem/1(Bogie) -> Bus Assignment/4  "Bogie"
  BogieGauges/1 -> Subsystem/1(BCPressure)

== system PneumaticsSystem/PneumaticsPerVehicle/PneumaticsSystem/MainReservoirSystem ==
  ControlStates : Inport
  ElectricalSignals : Inport  Port=2
  MRPUpPressure : Inport  Port=3
  MRPDownPressure : Inport  Port=4
  MRPUpConnection : Inport  Port=5
  MRPDownConnection : Inport  Port=6
  Coupled : Inport  Port=7
  MRPToAuxR : Inport  Port=8
  MRPToASR : Inport  Port=9
  MRPToBSR : Inport  Port=10
  Bus Creator : BusCreator  Inputs=3
  Bus Creator1 : BusCreator  Inputs=2
  Bus Selector : BusSelector  OutputSignals=MainCompressorOn
  Bus Selector3 : BusSelector  OutputSignals=MainAirSupplyIsolationCock,MainReservoirIsolationCock,MainReservoirDrainCock
  Bus Selector4 : BusSelector  OutputSignals=Pneumatics.Equipment.HasMainReservoir
  MainReservoir : Subsystem  mask{ResetPressure=Prm_PneumaticsSystem.MainReservoir.ResetPressure, MaxPressure=Prm_PneumaticsSystem.MainReservoir.MaxPressure, Volume=Prm_PneumaticsSystem.MainReservoir.Volume, PressureSwitchON=Prm_PneumaticsSystem.MainReservoir.SwitchONPressure, PressureSwitchOFF=Prm_PneumaticsSystem.MainReservoir.SwitchOFFPressure, CompMassFlow=Prm_PneumaticsSystem.MainReservoir.CompressorMassFlowRate, BlowOffON=Prm_PneumaticsSystem.MainReservoir.BlowOffONPressure, BlowOffOFF=Prm_PneumaticsSystem.MainReservoir.BlowOffOFFPressure}
      mask prompts: ResetPressure "Reset Pressure [Pa]"; MaxPressure "Max Pressure [Pa]"; Volume "Reservoir Volume [m^3]"; PressureSwitchON "Pressure Switch ON Point [Pa]"; PressureSwitchOFF "Pressure Switch OFF Point [Pa]"; CompMassFlow "Compressor Mass Flow Rate [kg/s]"; BlowOffON "Blow Off Valve ON Point [Pa]"; BlowOffOFF "Blow Off Valve OFF Point [Pa]"
  MainReservoirPipe : Subsystem  mask{ResetPressure=Prm_PneumaticsSystem.MainReservoirPipe.ResetPressure, PressureSwitchON=Prm_PneumaticsSystem.MainReservoirPipe.SwitchONPressure, PressureSwitchOFF=Prm_PneumaticsSystem.MainReservoirPipe.SwitchOFFPressure}
      mask prompts: ResetPressure "Reset Pressure [Pa]"; PressureSwitchON "Pressure Switch ON Point [Pa]"; PressureSwitchOFF "Pressure Switch OFF Point [Pa]"
  Unit Delay : UnitDelay  SampleTime=-1  HasFrameUpgradeWarning=on
  MRSystemPressures : Outport
  MRPPressureGauge : Outport  Port=2
  PressureSwitches : Outport  Port=3
  wires:
  MRPToBSR/1 -> MainReservoirPipe/5(MRPToBRFlowRate)
  MRPUpPressure/1 -> MainReservoirPipe/1(MRPUpPressure)
  MRPDownPressure/1 -> MainReservoirPipe/2(MRPDownPressure)
  MRPUpConnection/1 -> MainReservoirPipe/3(MRPUpConnection)
  MRPDownConnection/1 -> MainReservoirPipe/4(MRPDownConnection)
  MainReservoirPipe/1(MRPPressure) -> MainReservoir/5(MRPPressure), Bus Creator1/2  "MainReservoirPipePressure"
  MainReservoir/1(MRPressure) -> Bus Creator1/1  "MainReservoirPressure"
  MainReservoirPipe/3(MRPPressureSwitch) -> Bus Creator/2  "MainReservoirPipePressureSwitch"
  Bus Creator/1 -> PressureSwitches/1
  Bus Creator1/1 -> MRSystemPressures/1  "MRSystemPressures"
  MainReservoir/2(MRPressureSwitch) -> Bus Creator/1  "MainReservoirPressureSwitch"
  Bus Selector/1 -> MainReservoir/1(CompressorRunning)  "<MainCompressorOn>"
  ControlStates/1 -> Bus Selector3/1
  Bus Selector3/1 -> MainReservoir/2(AirSupplyIsolationCock)  "<MainAirSupplyIsolationCock>"
  Bus Selector3/2 -> MainReservoir/3(MainReservoirIsolationCock)  "<MainReservoirIsolationCock>"
  Bus Selector3/3 -> MainReservoir/4(MainReservoirDrainCock)  "<MainReservoirDrainCock>"
  ElectricalSignals/1 -> Bus Selector/1
  MainReservoirPipe/2(MRPPressureGauge) -> MRPPressureGauge/1
  [VehicleConfig] -> Bus Selector4/1
  Bus Selector4/1 -> MainReservoir/Enable  "<HasMainReservoir>"
  [Reset] -> MainReservoir/7(Reset)
  MainReservoirPipe/4(MRPS_TractionCutout) -> Bus Creator/3  "MRPS_TractionCutout"
  MainReservoir/3(MRPToMRFlow) -> Unit Delay/1
  Unit Delay/1 -> MainReservoirPipe/8(MRPToMRFlowRate)
  MRPToAuxR/1 -> MainReservoirPipe/7(MRPToAuxRFlowRate)
  MRPToASR/1 -> MainReservoirPipe/6(MRPToAirSuspFlowRate)
  Coupled/1 -> MainReservoir/6(Coupled)

== system PneumaticsSystem/PneumaticsPerVehicle/PneumaticsSystem/OutputMapping ==
  Axle : Inport
  PressureTransducers : Inport  Port=2
  Debug : Inport  Port=3
  Audio : Inport  Port=4
  PressureGauges : Inport  Port=5
  PressureSwitches : Inport  Port=6
  FaultMessages : Inport  Port=7
  Bus Creator : BusCreator  Inputs=7  OutDataTypeStr=Bus: BD_PneumaticsSystem_Out_Vehicle  NonVirtualBus=on
      settings: InheritFromInputs=off
  VehicleOut : Outport
  wires:
  Bus Creator/1 -> VehicleOut/1
  PressureSwitches/1 -> Bus Creator/5
  PressureGauges/1 -> Bus Creator/4
  Debug/1 -> Bus Creator/3
  Audio/1 -> Bus Creator/2
  PressureTransducers/1 -> Bus Creator/6
  Axle/1 -> Bus Creator/1
  FaultMessages/1 -> Bus Creator/7  "TCMS"

== system PneumaticsSystem/PneumaticsPerVehicle/PneumaticsSystem/PressuresMapping ==
  BogiePressures : Inport
  MRSystemPressures : Inport  Port=2
  PantoSystemPressures : Inport  Port=3
  BrakeReservoirPressure : Inport  Port=4
  Bus Assignment : BusAssignment  AssignedSignals=BrakeReservoirPressure,MainReservoirPressure,MainReservoirPipePressure,AuxiliaryReservoirPressure,PantographCylinderPressure,VCBCylinderPressure,Bogie
  Bus Selector1 : BusSelector  OutputSignals=MainReservoirPressure,MainReservoirPipePressure
  Bus Selector2 : BusSelector  OutputSignals=AuxiliaryReservoirPressure,PantographCylinderPressure,VCBCylinderPressure
  Constant : Constant  Value=0  OutDataTypeStr=Bus: BD_PneumaticsSystem_Out_Vehicle_Debug
  PressuresOut : Outport
  wires:
  MRSystemPressures/1 -> Bus Selector1/1
  PantoSystemPressures/1 -> Bus Selector2/1
  Bus Assignment/1 -> PressuresOut/1  "Debug"
  Bus Selector1/2 -> Bus Assignment/4  "<MainReservoirPipePressure>"
  Bus Selector2/1 -> Bus Assignment/5  "<AuxiliaryReservoirPressure>"
  Constant/1 -> Bus Assignment/1
  Bus Selector1/1 -> Bus Assignment/3  "<MainReservoirPressure>"
  Bus Selector2/2 -> Bus Assignment/6  "<PantographCylinderPressure>"
  BrakeReservoirPressure/1 -> Bus Assignment/2
  BogiePressures/1 -> Bus Assignment/8
  Bus Selector2/3 -> Bus Assignment/7  "<VCBCylinderPressure>"

== system PneumaticsSystem/PneumaticsPerVehicle/PneumaticsSystem/Subsystem1 ==
  PneuCoupled : Inport
  Add Constant : Bias  Bias=-1
  Bus Selector2 : BusSelector  OutputSignals=Common.Orientation,Pneumatics.Equipment.HasDriverCab
  CouplerNumber : Selector  InputPortWidth=2  IndexOptions=Index vector (dialog)  Indices=2  OutputSizes=1
  CouplerNumber1 : Selector  InputPortWidth=2  IndexOptions=Index vector (dialog)  Indices=1  OutputSizes=1
  Logical Operator1 : Logic  AllPortsSameDT=off  OutDataTypeStr=boolean
  Switch : Switch  Criteria=u2 > Threshold
  Coupled : Outport
  wires:
  Add Constant/1 -> Switch/2
  Bus Selector2/1 -> Add Constant/1  "<Orientation>"
  Logical Operator1/1 -> CouplerNumber1/1, CouplerNumber/1
  CouplerNumber1/1 -> Switch/3
  CouplerNumber/1 -> Switch/1
  Switch/1 -> Coupled/1
  PneuCoupled/1 -> Logical Operator1/2
  [VehicleConfig] -> Bus Selector2/1
  Bus Selector2/2 -> Logical Operator1/1  "<HasDriverCab>"

== system PneumaticsSystem/PneumaticsPerVehicle/PneumaticsSystem/SwitchesMapping ==
  BogieSwitches : Inport
  AuxSwitches : Inport  Port=2
  BrakeReservoirSwitch : Inport  Port=3
  MainReservoirSwitches : Inport  Port=4
  Bus Assignment : BusAssignment  AssignedSignals=BrakeReservoirPressureSwitch,MainReservoirPressureSwitch,MainReservoirPipePressureSwitch,MRPS_TractionCutout,HornHighPressureSwitch,HornLowPressureSwitch,AuxiliaryReservoirPressureSwitch,PS3,PS2,VCBPressureSwitch,Bogie
  Bus Selector : BusSelector  OutputSignals=HornLowPressureSwitch,HornHighPressureSwitch
  Bus Selector1 : BusSelector  OutputSignals=MainReservoirPressureSwitch,MainReservoirPipePressureSwitch,MRPS_TractionCutout
  Bus Selector3 : BusSelector  OutputSignals=AuxiliaryReservoirPressureSwitch,PS3,ORDPressureSwitch,VCBPressureSwitch
  Bus Selector4 : BusSelector  OutputSignals=HornPressureSwitches,PantoSystemPressureSwitches
  Constant : Constant  Value=0  OutDataTypeStr=Bus: BD_PneumaticsSystem_Out_Vehicle_Switches
  SwitchesOut : Outport
  wires:
  MainReservoirSwitches/1 -> Bus Selector1/1
  BrakeReservoirSwitch/1 -> Bus Assignment/2
  BogieSwitches/1 -> Bus Assignment/12
  AuxSwitches/1 -> Bus Selector4/1
  Bus Selector4/2 -> Bus Selector3/1  "<PantoSystemPressureSwitches>"
  Bus Selector4/1 -> Bus Selector/1  "<HornPressureSwitches>"
  Constant/1 -> Bus Assignment/1
  Bus Assignment/1 -> SwitchesOut/1  "PressureSwitches"
  Bus Selector/2 -> Bus Assignment/7  "<HornHighPressureSwitch>"
  Bus Selector3/1 -> Bus Assignment/8  "<AuxiliaryReservoirPressureSwitch>"
  Bus Selector3/2 -> Bus Assignment/9  "<PS3>"
  Bus Selector/1 -> Bus Assignment/6  "<HornLowPressureSwitch>"
  Bus Selector1/1 -> Bus Assignment/3  "<MainReservoirPressureSwitch>"
  Bus Selector1/2 -> Bus Assignment/4  "<MainReservoirPipePressureSwitch>"
  Bus Selector3/4 -> Bus Assignment/11  "<VCBPressureSwitch>"
  Bus Selector1/3 -> Bus Assignment/5  "<MRPS_TractionCutout>"
  Bus Selector3/3 -> Bus Assignment/10  "<ORDPressureSwitch>"

== system PneumaticsSystem/PneumaticsPerVehicle/PneumaticsSystem/TCMSMapping ==
  TCMSBogie : Inport
  Bus Creator5 : BusCreator  Inputs=1  OutDataTypeStr=Bus: BD_PneumaticsSystem_Out_Vehicle_TCMS  NonVirtualBus=on
  TCMSOut : Outport
  wires:
  TCMSBogie/1 -> Bus Creator5/1  "Bogie"
  Bus Creator5/1 -> TCMSOut/1  "TCMSOut"

== system PneumaticsSystem/PneumaticsPerVehicle/PneumaticsSystem/TrandsducersMapping ==
  BCUPressureTransducers : Inport
  Bus Creator5 : BusCreator  Inputs=1  OutDataTypeStr=Bus: BD_PneumaticsSystem_Out_Vehicle_Transducers  NonVirtualBus=on
      settings: InheritFromInputs=off
  TransducersOut : Outport
  wires:
  Bus Creator5/1 -> TransducersOut/1  "PressureTransducers"
  BCUPressureTransducers/1 -> Bus Creator5/1  "Bogie"

== system PneumaticsSystem/PneumaticsPerVehicle/PneumaticsSystem/ASReservoir/Air SuspensionReservoir ==
  MRPPressure : Inport
  ASRIsolCock : Inport  Port=2
  ASRDrainCock : Inport  Port=3
  ASFlow : Inport  Port=4
  Reset : Inport  Port=5
  Preset : Inport  Port=6
  PresetVal : Inport  Port=7
  AirSuspensionReservoir : PneumaticLib/Limited Air Pressure Vessel  resetPrs=ResetPressure + PAtm
      settings: SourceProductName=Pneumatic
  Constant : Constant  Value=PAtm + MaxPressure
  FlowCalc : Subsystem
  Terminator : Terminator
  Unit Delay : UnitDelay  SampleTime=-1  HasFrameUpgradeWarning=on
  pAtm : Constant  Value=PAtm
  pAtm2 : Constant  Value=Volume
  ASPressure : Outport
  MRPToASR : Outport  Port=2
  wires:
  Preset/1 -> AirSuspensionReservoir/6
  PresetVal/1 -> AirSuspensionReservoir/7
  ASRDrainCock/1 -> FlowCalc/4(ASRDrainCock)
  ASFlow/1 -> FlowCalc/5(ASFlow)
  ASRIsolCock/1 -> FlowCalc/3(ASRIsolCock)
  AirSuspensionReservoir/2 -> Terminator/1
  AirSuspensionReservoir/1 -> Unit Delay/1, ASPressure/1
  FlowCalc/2(Flow) -> AirSuspensionReservoir/1
  Constant/1 -> AirSuspensionReservoir/3
  MRPPressure/1 -> FlowCalc/1(MRPressure)
  Unit Delay/1 -> FlowCalc/2(ASRPressure)
  Reset/1 -> AirSuspensionReservoir/5
  pAtm/1 -> AirSuspensionReservoir/4
  pAtm2/1 -> AirSuspensionReservoir/2
  FlowCalc/1(MRPToASR) -> MRPToASR/1

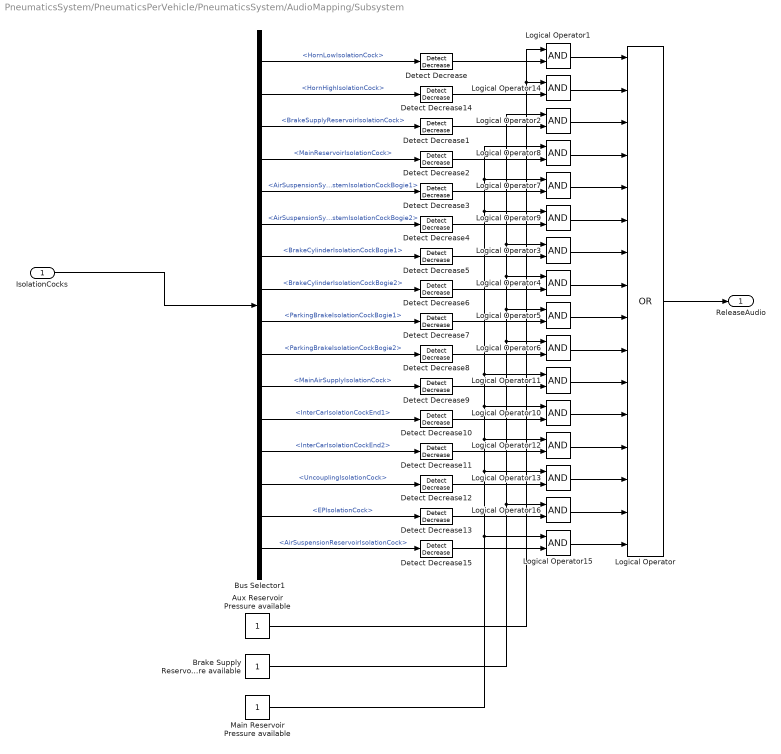
== system PneumaticsSystem/PneumaticsPerVehicle/PneumaticsSystem/AudioMapping/Subsystem ==
  IsolationCocks : Inport
  Aux Reservoir Pressure available : Constant
  Brake Supply Reservoir Pressure available : Constant
  Bus Selector1 : BusSelector  OutputSignals=HornLowIsolationCock,HornHighIsolationCock,BrakeSupplyReservoirIsolationCock,MainReservoirIsolationCock,AirSuspensionSystemIsolationCockBogie1,AirSuspensionSystemIsolationCockBogie2,BrakeCylinderIsolationCockBogie1,BrakeCylinderIsolationCockBogie2,ParkingBrakeIsolationCockBogie1,ParkingBrakeIsolationCockBogie2,MainAirSupplyIsolationCock,InterCarIsolationCockEnd1,InterCarIsolationCockEnd2,UncouplingIsolationCock,EPIsolationCock,AirSuspensionReservoirIsolationCock
  Detect Decrease{,1..15} (16 alike) : simulink/Logic and Bit Operations/Detect Decrease  vinit=0.0  OutDataTypeStr=boolean
  Logical Operator : Logic  Operator=OR  Inputs=16  AllPortsSameDT=off  OutDataTypeStr=boolean
  Logical Operator{1..16} (16 alike) : Logic  AllPortsSameDT=off  OutDataTypeStr=boolean
  Main Reservoir Pressure available : Constant
  ReleaseAudio : Outport
  wires:
  Bus Selector1/3 -> Detect Decrease1/1  "<BrakeSupplyReservoirIsolationCock>"
  Bus Selector1/7 -> Detect Decrease5/1  "<BrakeCylinderIsolationCockBogie1>"
  Bus Selector1/9 -> Detect Decrease7/1  "<ParkingBrakeIsolationCockBogie1>"
  Bus Selector1/4 -> Detect Decrease2/1  "<MainReservoirIsolationCock>"
  Bus Selector1/12 -> Detect Decrease10/1  "<InterCarIsolationCockEnd1>"
  Bus Selector1/1 -> Detect Decrease/1  "<HornLowIsolationCock>"
  Bus Selector1/14 -> Detect Decrease12/1  "<UncouplingIsolationCock>"
  Bus Selector1/11 -> Detect Decrease9/1  "<MainAirSupplyIsolationCock>"
  Bus Selector1/5 -> Detect Decrease3/1  "<AirSuspensionSystemIsolationCockBogie1>"
  Bus Selector1/10 -> Detect Decrease8/1  "<ParkingBrakeIsolationCockBogie2>"
  IsolationCocks/1 -> Bus Selector1/1
  Bus Selector1/8 -> Detect Decrease6/1  "<BrakeCylinderIsolationCockBogie2>"
  Bus Selector1/13 -> Detect Decrease11/1  "<InterCarIsolationCockEnd2>"
  Bus Selector1/6 -> Detect Decrease4/1  "<AirSuspensionSystemIsolationCockBogie2>"
  Logical Operator/1 -> ReleaseAudio/1
  Brake Supply Reservoir Pressure available/1 -> Logical Operator6/1, Logical Operator5/1, Logical Operator4/1, Logical Operator3/1, Logical Operator2/1, Logical Operator16/1
  Detect Decrease/1 -> Logical Operator1/2
  Detect Decrease1/1 -> Logical Operator2/2
  Detect Decrease2/1 -> Logical Operator8/2
  Detect Decrease3/1 -> Logical Operator7/2
  Detect Decrease4/1 -> Logical Operator9/2
  Detect Decrease6/1 -> Logical Operator4/2
  Detect Decrease5/1 -> Logical Operator3/2
  Detect Decrease7/1 -> Logical Operator5/2
  Detect Decrease8/1 -> Logical Operator6/2
  Detect Decrease10/1 -> Logical Operator10/2
  Detect Decrease9/1 -> Logical Operator11/2
  Detect Decrease11/1 -> Logical Operator12/2
  Detect Decrease12/1 -> Logical Operator13/2
  Aux Reservoir Pressure available/1 -> Logical Operator1/1, Logical Operator14/1
  Main Reservoir Pressure available/1 -> Logical Operator13/1, Logical Operator12/1, Logical Operator10/1, Logical Operator11/1, Logical Operator9/1, Logical Operator7/1, Logical Operator8/1, Logical Operator15/1
  Logical Operator1/1 -> Logical Operator/1
  Logical Operator2/1 -> Logical Operator/3
  Logical Operator8/1 -> Logical Operator/4
  Logical Operator7/1 -> Logical Operator/5
  Logical Operator9/1 -> Logical Operator/6
  Logical Operator3/1 -> Logical Operator/7
  Logical Operator5/1 -> Logical Operator/9
  Logical Operator4/1 -> Logical Operator/8
  Logical Operator12/1 -> Logical Operator/13
  Logical Operator6/1 -> Logical Operator/10
  Logical Operator11/1 -> Logical Operator/11
  Logical Operator10/1 -> Logical Operator/12
  Logical Operator13/1 -> Logical Operator/14
  Logical Operator14/1 -> Logical Operator/2
  Bus Selector1/2 -> Detect Decrease14/1  "<HornHighIsolationCock>"
  Detect Decrease14/1 -> Logical Operator14/2
  Bus Selector1/15 -> Detect Decrease13/1  "<EPIsolationCock>"
  Bus Selector1/16 -> Detect Decrease15/1  "<AirSuspensionReservoirIsolationCock>"
  Detect Decrease13/1 -> Logical Operator16/2
  Detect Decrease15/1 -> Logical Operator15/2
  Logical Operator16/1 -> Logical Operator/15
  Logical Operator15/1 -> Logical Operator/16

== system PneumaticsSystem/PneumaticsPerVehicle/PneumaticsSystem/AuxiliarySystems/AuxSystem ==
  ControlStates : Inport
  ElectricalSignals : Inport  Port=2
  MRSystemPressures : Inport  Port=3
  Faults : Inport  Port=4
  Reset : Inport  Port=5
  Enable : EnablePort
  Add : Sum
  AuxReservoir : Subsystem  mask{ResetPressure=Prm_PneumaticsSystem.AuxiliaryReservoir.ResetPressure, MaxPressure=Prm_PneumaticsSystem.AuxiliaryReservoir.MaxPressure, Volume=Prm_PneumaticsSystem.AuxiliaryReservoir.Volume, PressureSwitchON=Prm_PneumaticsSystem.AuxiliaryReservoir.SwitchONPressure, PressureSwitchOFF=Prm_PneumaticsSystem.AuxiliaryReservoir.SwitchOFFPressure, CompMassFlow=Prm_PneumaticsSystem.AuxiliaryReservoir.CompressorMassFlowRate, BlowOffON=Prm_PneumaticsSystem.AuxiliaryReservoir.BlowOffONPressure, BlowOffOFF=Prm_PneumaticsSystem.AuxiliaryReservoir.BlowOffOFFPressure}
      mask prompts: ResetPressure "Reset Pressure [Pa]"; MaxPressure "Max Pressure [Pa]"; Volume "Cylinder Volume [m^3]"; PressureSwitchON "Pressure Switch ON Point [Pa]"; PressureSwitchOFF "Pressure Switch OFF Point [Pa]"; CompMassFlow "Compessor Mass Flow Rate [kg/s]"; BlowOffON "Blow Off Valve ON Point [Pa]"; BlowOffOFF "Blow Off Valve OFF Point [Pa]"
  Bus Creator1 : BusCreator  Inputs=AuxiliaryReservoirPressureSwitch,PS3,VCBPressureSwitch,ORDPressureSwitch
  Bus Creator2 : BusCreator  Inputs=AuxiliaryReservoirPressure,PantographCylinderPressure,VCBCylinderPressure
  Bus Selector : BusSelector  OutputSignals=ORDPlunger,AuxiliaryCompressorIsolationCock,AuxiliaryReservoirIsolationCock,AuxiliaryReservoirDrainCock,PantographAirSupplyIsolationCock,VCBIsolationCock
  Bus Selector1 : BusSelector  OutputSignals=PantographRaiseValve,PantographEmergencyValve,AuxiliaryCompressorOn,VCBCloseCmd
  Bus Selector2 : BusSelector  OutputSignals=MainReservoirPipePressure
  Pantograph : Subsystem  mask{ResetPressure=Prm_PneumaticsSystem.Pantograph.ResetPressure, MaxPressure=Prm_PneumaticsSystem.Pantograph.MaxPressure, Volume=Prm_PneumaticsSystem.Pantograph.Volume, PressureSwitchON=Prm_PneumaticsSystem.Pantograph.SwitchONPressure, PressureSwitchOFF=Prm_PneumaticsSystem.Pantograph.SwitchOFFPressure, ORDPressureSwitchON=Prm_PneumaticsSystem.Pantograph.ORDSwitchONPressure, ORDPressureSwitchOFF=Prm_PneumaticsSystem.Pantograph.ORDSwitchOFFPressure}
      mask prompts: ResetPressure "Reset Pressure [Pa]"; MaxPressure "Max Pressure [Pa]"; Volume "Cylinder Volume [m^3]"; PressureSwitchON "Pressure Switch ON Point [Pa]"; PressureSwitchOFF "Pressure Switch OFF Point [Pa]"; ORDPressureSwitchON "Pressure Switch ON Point [Pa]"; ORDPressureSwitchOFF "Pressure Switch OFF Point [Pa]"
  Terminator : Terminator
  Unit Delay : UnitDelay  SampleTime=-1  HasFrameUpgradeWarning=on
  Unit Delay1 : UnitDelay  SampleTime=-1  HasFrameUpgradeWarning=on
  VCB : Subsystem  mask{ResetPressure=Prm_PneumaticsSystem.VCB.ResetPressure, MaxPressure=Prm_PneumaticsSystem.VCB.MaxPressure, PressureSwitchON=Prm_PneumaticsSystem.VCB.SwitchONPressure, PressureSwitchOFF=Prm_PneumaticsSystem.VCB.SwitchOFFPressure, Volume=Prm_PneumaticsSystem.VCB.Volume}
      mask prompts: ResetPressure "Reset Pressure [Pa]"; MaxPressure "Max Pressure [Pa]"; PressureSwitchON "Pressure Switch ON point [Pa]"; PressureSwitchOFF "Pressure Switch ON point [Pa]"; Volume "Cylinder Volume [m^3]"
  PantoSystemPressures : Outport
  PressureSwitches : Outport  Port=2
  MRPToAuxR : Outport  Port=3
  wires:
  Pantograph/2(PS3) -> Bus Creator1/2
  AuxReservoir/2(ARPressureSwitch) -> Bus Creator1/1
  Bus Creator1/1 -> PressureSwitches/1  "PantoSystemPressureSwitches"
  Bus Selector1/3 -> AuxReservoir/1(CompressorRunning)  "<AuxiliaryCompressorOn>"
  ElectricalSignals/1 -> Bus Selector1/1
  MRSystemPressures/1 -> Bus Selector2/1
  ControlStates/1 -> Bus Selector/1
  Bus Selector/2 -> AuxReservoir/3(AuxCompIsolCock)  "<AuxiliaryCompressorIsolationCock>"
  Bus Selector/5 -> Pantograph/3(PantoAirSupplyIsolCock)  "<PantographAirSupplyIsolationCock>"
  Pantograph/3(ARtoPCFlow) -> Unit Delay/1
  Pantograph/1(PCPressure) -> Bus Creator2/2
  Bus Creator2/1 -> PantoSystemPressures/1  "PantoSystemPressures"
  Bus Selector1/1 -> Pantograph/1(PanRaiseValve)  "<PantographRaiseValve>"
  Bus Selector1/2 -> Pantograph/2(PantoEmerValve)  "<PantographEmergencyValve>"
  Bus Selector/4 -> AuxReservoir/5(ARDrainCock)  "<AuxiliaryReservoirDrainCock>"
  Bus Selector/3 -> AuxReservoir/4(ARIsolCock)  "<AuxiliaryReservoirIsolationCock>"
  Reset/1 -> VCB/2(Reset1), AuxReservoir/7(Reset), Pantograph/5(Reset)
  VCB/1(VCBCylinderPressure) -> Bus Creator2/3
  VCB/2(VCBPressureSwitch) -> Bus Creator1/3
  Unit Delay/1 -> Add/1
  Unit Delay1/1 -> Add/2
  Add/1 -> AuxReservoir/6(ARtoPCandVCBFlow)  "ARtoPCandVCB Flow"
  VCB/3(ARtoVCB) -> Unit Delay1/1
  Bus Selector2/1 -> AuxReservoir/2(MRPPressure)  "<MainReservoirPipePressure>"
  Faults/1 -> Pantograph/6(Fault)
  AuxReservoir/1(ARPressure) -> Pantograph/4(ARPressure), Bus Creator2/1, VCB/1(ARPressure)
  AuxReservoir/3(MRPToAuxR) -> MRPToAuxR/1
  Bus Selector1/4 -> VCB/3(VCBC)  "<VCBCloseCmd>"
  Bus Selector/6 -> VCB/4(VCBIsolationCock)  "<VCBIsolationCock>"
  Pantograph/4(PS1) -> Terminator/1
  Pantograph/5(PS2) -> Bus Creator1/4
  Bus Selector/1 -> Pantograph/7(WVM2)  "<ORDPlunger>"
